simulink model "template_rotary_inverted_pendulum_2012b"  (R2012b)
settings: Solver=FixedStepDiscrete  SolverMode=SingleTasking  StartTime=0.0  StopTime=inf  FixedStep=0.005  RelTol=1e-3
undefined symbols (not defined in the file or in its folder): National_Instruments, PCI
libraries: rtwinlib x2, simulink_extras x2
settings Model: SimulationMode=external  ExtModeTrigDuration=200000  Creator=magudelo  LastModifiedBy=Mauricio
settings SolverCC: InsertRTBMode=Always
settings DataIOCC: SignalLoggingSaveFormat=ModelDataLogs
settings DebuggingCC: FcnCallInpInsideContextMsg=UseLocalSettings  StrictBusMsg=Warning
settings HardwareCC: ProdIntDivRoundTo=Zero  ProdEndianess=LittleEndian  ProdHWDeviceType=Generic->32-bit x86 compatible
settings RTWCC: SystemTargetFile=rtwin.tlc  TemplateMakefile=rtwin.tmf  Description=Real-Time Windows Target  ProcessScript=rtwin_make_rtw_hook  RTWCompilerOptimization=On
settings CodeAppCC: MaxIdLength=95
settings RTWinTargetCC: TargetLibSuffix=_rtwin.lib  TargetPreCompLibLocation=C:\MATLAB\R2012b\toolbox\rtw\targets\rtwin\lib\win64  CodeReplacementLibrary=ANSI_C  RTWinDir=C:/MATLAB/R2012b/toolbox/rtw/targets/rtwin  TargetArch=win64

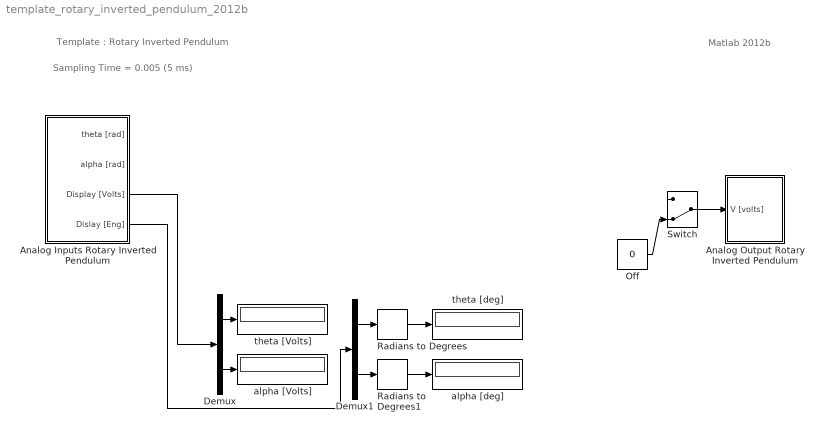
== system template_rotary_inverted_pendulum_2012b ==
  note: Matlab 2012b
  note: Sampling Time = 0.005 (5 ms)
  note: Template : Rotary Inverted Pendulum
  Analog Inputs Rotary Inverted Pendulum : Subsystem  mask(Analog Inputs. Rotary Inverted Pendulum){factor_theta=0.5959, offset_theta=-1.3, factor_alfa=0.3, offset_alfa=0.54}
      mask prompts: factor_theta "F_theta = Convertion factor from Volts to Radians (theta) :"; offset_theta "Off_theta = Offset for the angle of the arm (Volts):"; factor_alfa "F_alpha = Convertion Factor From Volts to Radians (alfa) :"; offset_alfa "Off_alpha = Offset for the angle of the rob (Volts) :"
      mask help:
      | Remember:
      |    Angle of the arm (theta) => channel ACH0
      |    Angle of the rod (alpha)    => channel ACH1
      |
      |   Angle of the arm  [rad] = F_theta * ( Angle of the arm [v]  + off_theta )
      |   Angle of the rod [rad] = F_alpha * ( Angle of the rod [v] + off_alpha )
  Analog Output Rotary Inverted Pendulum : Subsystem  mask(Analog Output - Rotary Inverted Pendulum){}
      mask help:
      | Remember
      |    AO 0 => Power Amplifier + Motor
  Demux : Demux  Outputs=2
  Demux1 : Demux  Outputs=2
  Off : Constant  Value=0
  Radians to Degrees : simulink_extras/Transformations/Radians to Degrees
  Radians to Degrees1 : simulink_extras/Transformations/Radians to Degrees
  "Switch  " : ManualSwitch  CurrentSetting=0
  alpha [Volts] : Display
      settings: SampleTime=0.25
  alpha [deg] : Display
      settings: SampleTime=0.25
  theta [Volts] : Display
      settings: SampleTime=0.25
  theta [deg] : Display
      settings: SampleTime=0.25
  wires:
  Demux/1 -> theta [Volts]/1
  Demux/2 -> alpha [Volts]/1
  Analog Inputs Rotary Inverted Pendulum/3(Display [Volts]) -> Demux/1
  Analog Inputs Rotary Inverted Pendulum/4(Dislay [Eng]) -> Demux1/1
  Off/1 -> "Switch  "/2
  "Switch  "/1 -> Analog Output Rotary Inverted Pendulum/1(V [volts])
  Demux1/1 -> Radians to Degrees/1
  Radians to Degrees/1 -> theta [deg]/1
  Demux1/2 -> Radians to Degrees1/1
  Radians to Degrees1/1 -> alpha [deg]/1

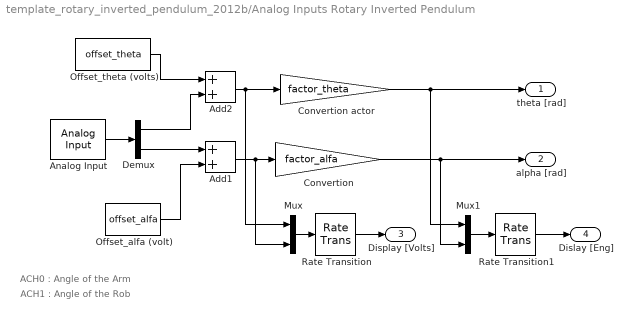
== system template_rotary_inverted_pendulum_2012b/Analog Inputs Rotary Inverted Pendulum ==
  note: ACH1 : Angle of the Rob
  note: ACH0 : Angle of the Arm
  Add1 : Sum
  Add2 : Sum
  Analog Input : rtwinlib/Analog Input  SampleTime=0.005  MaxMissedTicks=10  ShowMissedTicks=off  YieldWhenWaiting=off  DrvName=National_Instruments/PCI-6014  DrvAddress=1  DrvOptions=[1 0 0 0 0 0]  Channels=[1 2]  RangeMode=1  VoltRange=1  DataType=1
      settings: AttributesFormatString=National Instruments\nPCI-6014 [1h]
  "Convertion " : Gain  Gain=factor_alfa
  Convertion actor : Gain  Gain=factor_theta
  Demux : Demux  Outputs=2
  Mux : Mux  Inputs=2
  Mux1 : Mux  Inputs=2
  Offset_alfa (volt) : Constant  Value=offset_alfa
  Offset_theta (volts) : Constant  Value=offset_theta
  Rate Transition : RateTransition  OutPortSampleTime=0.25
  Rate Transition1 : RateTransition  OutPortSampleTime=0.25
  theta [rad] : Outport
  alpha [rad] : Outport  Port=2
  Display [Volts] : Outport  Port=3
  Dislay [Eng] : Outport  Port=4
  wires:
  Rate Transition1/1 -> Dislay [Eng]/1
  Mux1/1 -> Rate Transition1/1
  Rate Transition/1 -> Display [Volts]/1
  Mux/1 -> Rate Transition/1
  "Convertion "/1 -> Mux1/2, alpha [rad]/1
  Add1/1 -> Mux/2, "Convertion "/1
  Offset_alfa (volt)/1 -> Add1/2
  Demux/2 -> Add1/1
  Convertion actor/1 -> Mux1/1, theta [rad]/1
  Offset_theta (volts)/1 -> Add2/1
  Add2/1 -> Mux/1, Convertion actor/1
  Demux/1 -> Add2/2
  Analog Input/1 -> Demux/1

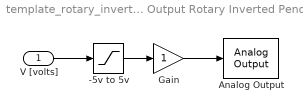
== system template_rotary_inverted_pendulum_2012b/Analog Output Rotary Inverted Pendulum ==
  V [volts] : Inport
  -5v to 5v : Saturate  UpperLimit=5  LowerLimit=-5
  Analog Output : rtwinlib/Analog Output  SampleTime=0.005  MaxMissedTicks=10  ShowMissedTicks=off  YieldWhenWaiting=off  DrvName=National_Instruments/PCI-6014  DrvAddress=1  DrvOptions=[1 0 0 0 0 0]  Channels=1  RangeMode=1  VoltRange=1  InitialValue=0  FinalValue=0
      settings: AttributesFormatString=National Instruments\nPCI-6014 [1h]
  Gain : Gain
  wires:
  V [volts]/1 -> -5v to 5v/1
  -5v to 5v/1 -> Gain/1
  Gain/1 -> Analog Output/1
